simulink model "roll_pitch_yaw"  (Simulink 7.4)
settings: Solver=ode45  StartTime=0.0  StopTime=6000  RelTol=1e-3
libraries: aausat3_lib x15
settings Model: Creator=kasperv  LastModifiedBy=Administrator

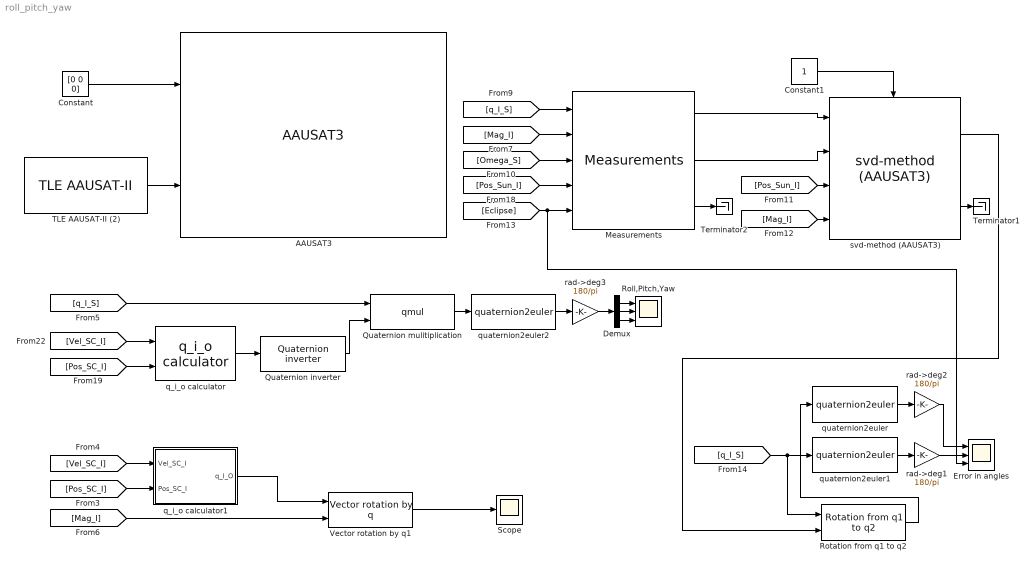
== system roll_pitch_yaw ==
  AAUSAT3 : aausat3_lib/AAUSAT3  SystemSampleTime=-1  r_com_s=[0.049073,0.048909,0.042976]  sat_temp_start=293.15  mass_sc=0.957820  Dim=[0.1,0.1,0.11]  inertia_c=[0.0017464,0.0022092,0.0022388]  init_jd=2455153.1954318+0.035  q_s_c=[-0.020656,0.71468,-0.007319,0.6991]  q_init_I_S=[0 0 0 1]  w_init_s=[0.02,0.02,0.02]  Cd=2  rho=5e-14  solar_m_flux=4.5565e-6  solar_absorb_coeff=1.5  theta_e=65  refldata=load('lib/AlbedoToolbox-1.0/refl_data/2005/ga050101-051231')  redfac=1  Ts=1  enable_sensor_emulation=on  enable_env_disturbance=on
  Constant : Constant  Value=[0 0 0]  OutDataType=fixdt(1, 16)  OutScaling=2^0
  Constant1 : Constant  OutDataType=fixdt(1, 16)  OutScaling=2^0
  Demux : Demux  Outputs=3
  Error in angles : Scope  NumInputPorts=3
      settings: TimeRange=6000  YMin=-27.5~-80~-1  YMax=17.5~140~1  SaveName=ScopeData2  SampleInput=on  SampleTime=1
  Measurements : aausat3_lib/Sensor Emulation/Measurements  SystemSampleTime=-1  s_freq_mag=1  noise_mag=3  bias_mag=[2000 4000 0]  heading_mag=0  tilt_mag=0  s_freq_sun=1  noise_sun=3.33  bias_sun=[0 0]  nr_sample_sun=1  s_freq_gyro=1  noise_gyro=0.2  bias_gyro=[-0.2 -0.2 -0.2]  heading_gyro=0  tilt_gyro=0
  Quaternion inverter : aausat3_lib/Math Utilities/Quaternion operations/Quaternion inverter  SystemSampleTime=-1
  Quaternion mulitiplication : S-Function  FunctionName=qmul  EnableBusSupport=off
  Roll,Pitch,Yaw : Scope  NumInputPorts=3
      settings: TimeRange=48000  YMin=86.5~-38~175.7  YMax=88.1~-35~177.7  SampleInput=on  SampleTime=1
  Rotation from q1 to q2 : aausat3_lib/Math Utilities/Quaternion operations/Rotation from q1 to q2  SystemSampleTime=-1
  Scope : Scope
      settings: YMin=-2.2e-005  YMax=-1e-006
  TLE AAUSAT-II (2) : aausat3_lib/Orbit and Ephemeris/TLE AAUSAT-II  SystemSampleTime=-1  satname='AAUSAT-II'  JulianDay=09321.69542252  xndt2o=0.00000555  xndd6o=0.0  bstar=.76898e-4  xincl=97.9251  xnodeo=24.1597  eo=0.0014245  omegao=254.1774  xmo=105.7862  xno=14.81823818  ts=1
  Terminator1 : Terminator
  Terminator2 : Terminator
  Vector rotation by q1 : aausat3_lib/Math Utilities/Quaternion operations/Vector rotation by q  SystemSampleTime=-1
  q_i_o calculator : aausat3_lib/Math Utilities/q_i_o calculator  SystemSampleTime=-1
  q_i_o calculator1 : Subsystem  AncestorBlock=aausat3_lib/Math Utilities/q_i_o calculator
  quaternion2euler : aausat3_lib/Math Utilities/Quaternion operations/quaternion2euler  SystemSampleTime=-1
  quaternion2euler1 : aausat3_lib/Math Utilities/Quaternion operations/quaternion2euler  SystemSampleTime=-1
  quaternion2euler2 : aausat3_lib/Math Utilities/Quaternion operations/quaternion2euler  SystemSampleTime=-1
  rad->deg1 : Gain  Gain=180/pi  ParameterDataType=fixdt(1, 16)  ParameterScaling=2^0  OutDataType=fixdt(1, 16)  OutScaling=2^0
  rad->deg2 : Gain  Gain=180/pi  ParameterDataType=fixdt(1, 16)  ParameterScaling=2^0  OutDataType=fixdt(1, 16)  OutScaling=2^0
  rad->deg3 : Gain  Gain=180/pi  ParameterDataType=fixdt(1, 16)  ParameterScaling=2^0  OutDataType=fixdt(1, 16)  OutScaling=2^0
  svd-method (AAUSAT3) : aausat3_lib/ADS/svd-method (AAUSAT3)  SystemSampleTime=-1  f_sample=10  weigth_a=[1/0.0034 1/0.0027]
      link override Weights: Value=weigth_a
  wires:
  q_i_o calculator/1 -> Quaternion inverter/1
  Quaternion inverter/1 -> Quaternion mulitiplication/2
  Quaternion mulitiplication/1 -> quaternion2euler2/1
  quaternion2euler2/1 -> rad->deg3/1
  rad->deg3/1 -> Demux/1
  Demux/1 -> Roll,Pitch,Yaw/1
  Demux/2 -> Roll,Pitch,Yaw/2
  Demux/3 -> Roll,Pitch,Yaw/3
  [q_I_S] -> Quaternion mulitiplication/1
  [Vel_SC_I] -> q_i_o calculator/1
  [Pos_SC_I] -> q_i_o calculator/2
  TLE AAUSAT-II (2)/1 -> AAUSAT3/2
  Constant/1 -> AAUSAT3/1
  [Vel_SC_I] -> q_i_o calculator1/1(Vel_SC_I)
  [Pos_SC_I] -> q_i_o calculator1/2(Pos_SC_I)
  [Mag_I] -> Vector rotation by q1/2
  q_i_o calculator1/1(q_I_O) -> Vector rotation by q1/1
  Vector rotation by q1/1 -> Scope/1
  [q_I_S] -> Measurements/1
  [Mag_I] -> Measurements/2
  [Omega_S] -> Measurements/3
  [Eclipse] -> Measurements/5, Error in angles/3
  [Pos_Sun_I] -> Measurements/4
  Constant1/1 -> svd-method (AAUSAT3)/Enable
  Measurements/1 -> svd-method (AAUSAT3)/1
  Measurements/2 -> svd-method (AAUSAT3)/2
  Measurements/3 -> Terminator2/1
  [Pos_Sun_I] -> svd-method (AAUSAT3)/3
  [Mag_I] -> svd-method (AAUSAT3)/4
  [q_I_S] -> Rotation from q1 to q2/1, quaternion2euler1/1
  Rotation from q1 to q2/1 -> quaternion2euler/1
  rad->deg2/1 -> Error in angles/1
  rad->deg1/1 -> Error in angles/2
  quaternion2euler1/1 -> rad->deg1/1
  quaternion2euler/1 -> rad->deg2/1
  svd-method (AAUSAT3)/1 -> Rotation from q1 to q2/2
  svd-method (AAUSAT3)/2 -> Terminator1/1

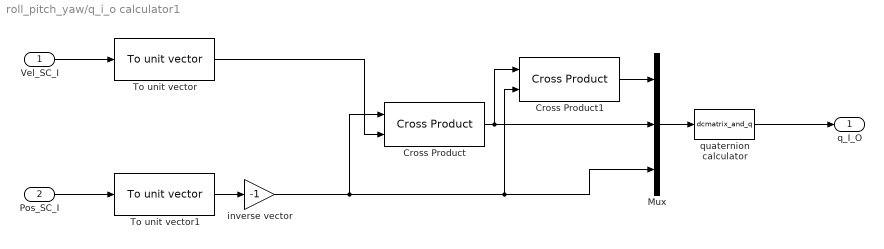
== system roll_pitch_yaw/q_i_o calculator1 ==
  Vel_SC_I : Inport  OutDataType=sfix(16)  OutScaling=2^0
  Pos_SC_I : Inport  Port=2  OutDataType=sfix(16)  OutScaling=2^0
  Cross Product : aausat3_lib/Math Utilities/Vector operations/Cross Product  SystemSampleTime=-1
  Cross Product1 : aausat3_lib/Math Utilities/Vector operations/Cross Product  SystemSampleTime=-1
  Mux : Mux  Inputs=3
  To unit vector : aausat3_lib/Math Utilities/Vector operations/To unit vector  SystemSampleTime=-1
  To unit vector1 : aausat3_lib/Math Utilities/Vector operations/To unit vector  SystemSampleTime=-1
  inverse vector : Gain  Gain=-1  ParameterDataType=fixdt(1, 16)  ParameterScaling=2^0  OutDataType=fixdt(1, 16)  OutScaling=2^0
  quaternion calculator : MATLABFcn  Description=|  MATLABFcn=dcmatrix_and_q
      | Direction cosine matrix computation.                               
      | O1,O2,O3 are the three unit vectors representing the axes of the   
      | rotated coordinate system given in the reference coordinate system.
  q_I_O : Outport  OutDataType=sfix(16)  OutScaling=2^0
  wires:
  To unit vector/1 -> Cross Product/2
  Mux/1 -> quaternion calculator/1
  To unit vector1/1 -> inverse vector/1
  inverse vector/1 -> Cross Product/1, Mux/3, Cross Product1/2
  Vel_SC_I/1 -> To unit vector/1
  Pos_SC_I/1 -> To unit vector1/1
  quaternion calculator/1 -> q_I_O/1
  Cross Product/1 -> Mux/2, Cross Product1/1
  Cross Product1/1 -> Mux/1
